simulink model "built_in_model"  (R2024b)
settings: Solver=VariableStepAuto  StartTime=0.0  StopTime=10.0  RelTol=1e-3
values from neighbouring files (symbols this model uses):
  B = 0.0015    [Test_script.m]
  J = 0.015    [Test_script.m]
  Llr = 12e-3    (= 0.012)    [Test_script.m]
  Lls = 12e-3    (= 0.012)    [Test_script.m]
  P = 2    [Test_script.m]
  r_r = 0.9    [Test_script.m]
  r_s = 1.2    [Test_script.m]
undefined symbols (not defined in the file or in its folder): Tl
libraries: spsVoltageMeasurementLib x3, spsAsynchronousMachineSIUnitsLib x1, spsThreePhaseSourceLib x1
settings Model: Creator=mafur  LastModifiedBy=mafur

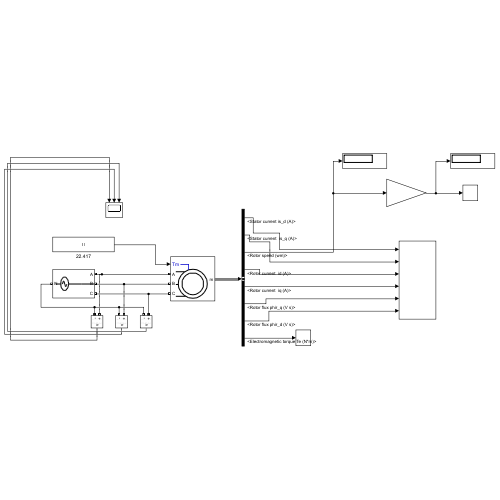
[thumbnail: Simulink's stored preview of the top-level diagram]
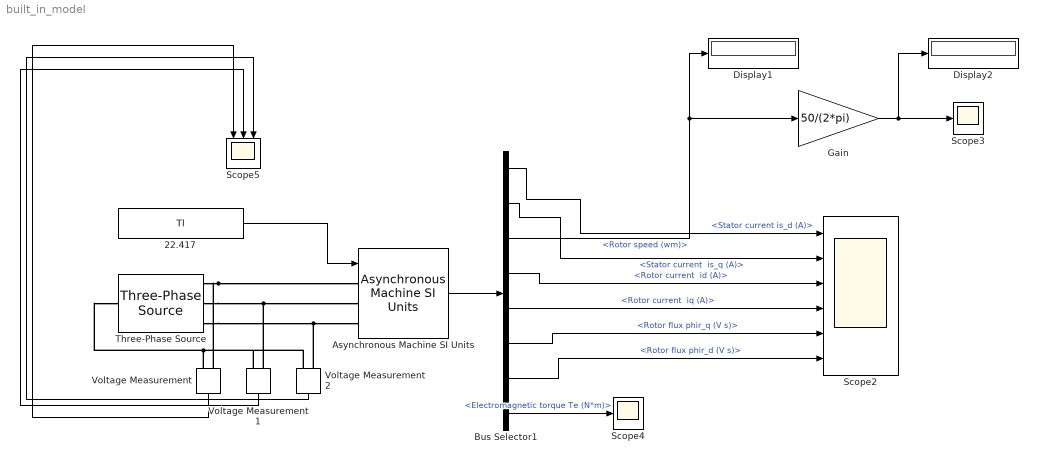
== system built_in_model ==
  22.417 : Constant  Value=Tl
  Asynchronous Machine SI Units : spsAsynchronousMachineSIUnitsLib/Asynchronous Machine SI Units  RotorType=Squirrel-cage  PresetModel=No  MechanicalLoad=Torque Tm  ShowDetailedParameters=on  ReferenceFrame=Stationary  Units=SI  MeasurementBus=off  NominalParameters=[1.845e+04 230 50]  VoltageRatio=1  Stator=[r_s Lls]  Rotor=[r_r Llr]  Cage1=[0.4155 0.002066]  Cage2=[0.4168 0.0003495]  Lm=LM  Mechanical=[J B P/2]  PolePairs=2  InitialConditions=[1 0 0 0 0 0 -120 120]  SimulateSaturation=off  Saturation=[14.03593122, 27.81365428, 53.79336849, 72.68890987, 97.98006896, 148.6815601, 215.7428561, 302.9841135, 428.7778367 ; 230, 322, 414, 460, 506, 552, 598, 644, 690]  LoadFlowParameters=1492000  TsPowergui=0  TsBlock=-1  IterativeModel=Trapezoidal non iterative  IterativeDiscreteModel=Trapezoidal non iterative  Pmec=1.492e+006
  Bus Selector1 : BusSelector  OutputSignals="Stator measurements.Stator current is_d (A),Stator measurements.Stator current  is_q (A),Mechanical.Rotor speed (wm),Rotor measurements.Rotor current  id (A),Rotor measurements.Rotor current  iq (A),Rotor measurements.Rotor flux phir_q (V s),Rotor measurements.Rotor flux phir_d (V s),Mechanical.Electromagnetic torque Te (N*m)"
  Display1 : Display
  Display2 : Display
  Gain : Gain  Gain=50/(2*pi)
  Scope2 : Scope  NumInputPorts=6
  Scope3 : Scope
  Scope4 : Scope
  Scope5 : Scope  NumInputPorts=3
  Three-Phase Source : spsThreePhaseSourceLib/Three-Phase Source  InternalConnection=Yn  VoltagePhases=off  Voltage=400  PhaseAngle=0  Voltage_phases=[25e3 25e3 25e3]/sqrt(3)  PhaseAngles_phases=[0 -120 +120]  Frequency=50  NonIdealSource=off  SpecifyImpedance=off  Resistance=0.8929  Inductance=16.58e-3  ShortCircuitLevel=100e6  BaseVoltage=25e3  XRratio=7  BusType=swing  Pref=10e3  Qref=0  Prefabc=[10e3, 10e3, 10e3]  Qrefabc=[0, 0, 0]  Qmin=-inf  Qmax=inf
  Voltage Measurement : spsVoltageMeasurementLib/Voltage Measurement  PhasorSimulation=off  OutputType=Complex  PSBequivalent=0
  Voltage Measurement1 : spsVoltageMeasurementLib/Voltage Measurement  PhasorSimulation=off  OutputType=Complex  PSBequivalent=0
  Voltage Measurement2 : spsVoltageMeasurementLib/Voltage Measurement  PhasorSimulation=off  OutputType=Complex  PSBequivalent=0
  wires:
  Voltage Measurement/1 -> Scope5/1
  Voltage Measurement2/1 -> Scope5/3
  Voltage Measurement1/1 -> Scope5/2
  Gain/1 -> Display2/1, Scope3/1
  Bus Selector1/7 -> Scope2/6  "<Rotor flux phir_d (V s)>"
  Asynchronous Machine SI Units/1 -> Bus Selector1/1
  Bus Selector1/8 -> Scope4/1  "<Electromagnetic torque Te (N*m)>"
  Bus Selector1/4 -> Scope2/3  "<Rotor current  id (A)>"
  Bus Selector1/3 -> Display1/1, Gain/1  "<Rotor speed (wm)>"
  22.417/1 -> Asynchronous Machine SI Units/1
  Bus Selector1/6 -> Scope2/5  "<Rotor flux phir_q (V s)>"
  Bus Selector1/2 -> Scope2/2  "<Stator current  is_q (A)>"
  Bus Selector1/5 -> Scope2/4  "<Rotor current  iq (A)>"
  Bus Selector1/1 -> Scope2/1  "<Stator current is_d (A)>"
  connections:
  Three-Phase Source/RConn3 -- Voltage Measurement2/LConn1 -- Asynchronous Machine SI Units/LConn3
  Voltage Measurement/LConn2 -- Voltage Measurement2/LConn2 -- Voltage Measurement1/LConn2 -- Three-Phase Source/LConn1
  Three-Phase Source/RConn2 -- Voltage Measurement1/LConn1 -- Asynchronous Machine SI Units/LConn2
  Three-Phase Source/RConn1 -- Asynchronous Machine SI Units/LConn1 -- Voltage Measurement/LConn1
